simulink model "sistema_termico"  (R2019b)
settings: Solver=VariableStepAuto  StartTime=0.0  StopTime=30  RelTol=1e-3
model workspace (MAT data in the model file):
  algo = 1
settings Model: EnablePacing=on  Creator=Fabian  LastModifiedBy=fmj.durango10

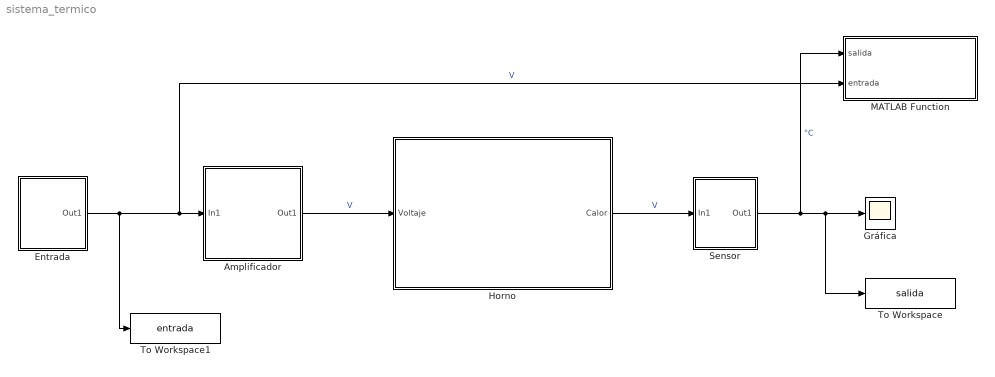
== system sistema_termico ==
  Amplificador : Subsystem
      mask Display: image('$imagefile'); % Use "Edit Image" on toolstrip to change.
  Entrada : Subsystem
      mask Display: image('$imagefile'); % Use "Edit Image" on toolstrip to change.
  Gráfica : Scope
  Horno : Subsystem
      mask Display: image('$imagefile'); % Use "Edit Image" on toolstrip to change.
  MATLAB Function : MATLAB Function  TreatAsAtomicUnit=on
  Sensor : Subsystem
      mask Display: image('$imagefile'); % Use "Edit Image" on toolstrip to change.
  To Workspace : ToWorkspace  VariableName=salida  SaveFormat=Timeseries  SampleTime=-1
  To Workspace1 : ToWorkspace  VariableName=entrada  SaveFormat=Timeseries  SampleTime=-1
  wires:
  Amplificador/1(Out1) -> Horno/1(Voltaje)  "V"
  Entrada/1(Out1) -> To Workspace1/1, MATLAB Function/2(entrada), Amplificador/1(In1)  "V"
  Horno/1(Calor) -> Sensor/1(In1)  "V"
  Sensor/1(Out1) -> MATLAB Function/1(salida), To Workspace/1, Gráfica/1  "°C"

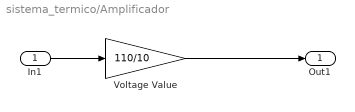
== system sistema_termico/Amplificador ==
  In1 : Inport
  Voltage Value : Gain  Gain=110/10
  Out1 : Outport
  wires:
  In1/1 -> Voltage Value/1
  Voltage Value/1 -> Out1/1

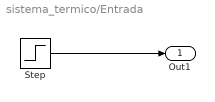
== system sistema_termico/Entrada ==
  Step : Step  Time=0  After=10  SampleTime=0
  Out1 : Outport
  wires:
  Step/1 -> Out1/1

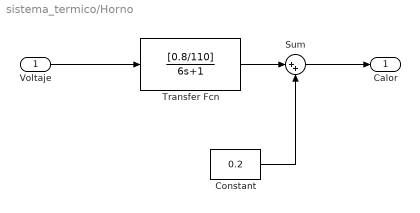
== system sistema_termico/Horno ==
  Voltaje : Inport
  Constant : Constant  Value=0.2  VectorParams1D=off
  Sum : Sum  Inputs=|++
  Transfer Fcn : TransferFcn  Numerator=[0.8/110]  Denominator=[6 1]
  Calor : Outport
  wires:
  Voltaje/1 -> Transfer Fcn/1
  Constant/1 -> Sum/2
  Transfer Fcn/1 -> Sum/1
  Sum/1 -> Calor/1

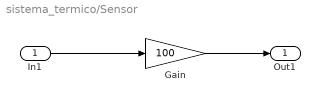
== system sistema_termico/Sensor ==
  In1 : Inport
  Gain : Gain  Gain=100
  Out1 : Outport
  wires:
  In1/1 -> Gain/1
  Gain/1 -> Out1/1

== matlab function sistema_termico/MATLAB Function ==
  data: salida input; entrada input
function fcn(salida, entrada)
if salida>100
    salida=100;
elseif salida<0
    salida=0;
end
if entrada>10
    entrada=10;
elseif entrada<0
    entrada=0;
end
clf

rectangle('Position',[0 0 10 7],'FaceColor',[1 1 1])
rectangle('Position',[1 1 4 3],'FaceColor',[138/255 139/255 137/255])
hold on
rectangle('Position',[1.7 1.5 2.9 2],'FaceColor',[255/255 255/255 (10-entrada)/10])
rectangle('Position',[1.2 0.8 0.2 0.2],'FaceColor',[0/255 0/255 0/255])
rectangle('Position',[4.6 0.8 0.2 0.2],'FaceColor',[0/255 0/255 0/255])
rectangle('Position',[1.3 2 0.2 0.8],'FaceColor',[0/255 0/255 0/255])
rectangle('Position',[4.4 2.7 1 0.1],'FaceColor',[32/255 126/255 138/255])
rectangle('Position',[5.4 2.4 1.5 0.7],'FaceColor',[32/255 126/255 138/255])
rectangle('Position',[5.5 2.5 1.3 0.5],'FaceColor',[255/255 255/255 255/255])

rectangle('Position',[7.85 3 0.8 salida*3/100],'FaceColor',[255/255 (100-salida)/80 0],'EdgeColor',[255/255 (100-salida)/80 0])
rectangle('Position',[7.5 2 1.5 1.5],'FaceColor',[255/255 (100-salida)/80 0],'EdgeColor',[255/255 (100-salida)/80 0],'Curvature',[1 1])
for i=0:12
    plot([7.4 7.6],[3.6+i*0.2 3.6+i*0.2],'Color','k')
end
text(6.6,3.6,'20 C')
text(6.6,6,' 100 C')

% text(2.1,1.9,'\it h_2=')
text(5.8,2.7,sprintf('%.2f',abs(salida)))
text(6.4,2.7,'C')
text(1,5.5,'\bf Sistema de primer orden','FontSize',16)


% title('Horno')
set(gcf, 'Position',  [300, 50, 800, 620])

hold off
axis off
axis([0 10 0 7])
